simulink model "Einfache_Zustandsrueckfuehrung_nichtlinear"  (R2021b)
settings: Solver=VariableStepAuto  StartTime=0.0  StopTime=3  FixedStep=1/1e6  RelTol=1e-3
undefined symbols (not defined in the file): C_buck, k_LMI_1, L_buck, S, T_c, x_Ruhe
settings Model: Creator=basti  LastModifiedBy=basti

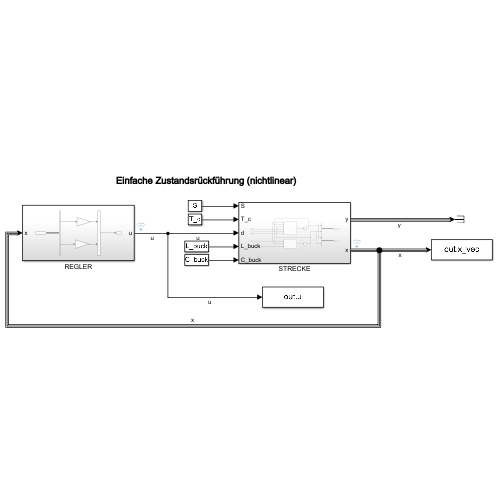
[thumbnail: Simulink's stored preview of the top-level diagram]
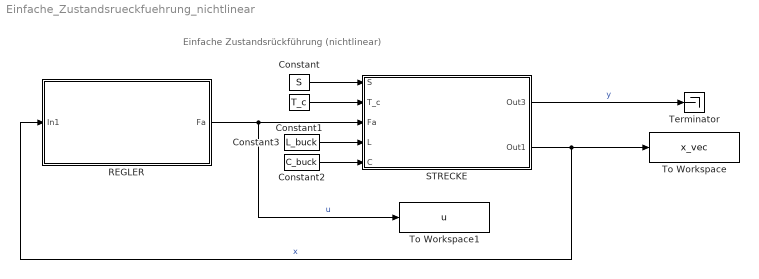
== system Einfache_Zustandsrueckfuehrung_nichtlinear ==
  note: Einfache Zustandsrückführung (nichtlinear)
  Constant : Constant  Value=S
  Constant1 : Constant  Value=T_c
  Constant2 : Constant  Value=C_buck
  Constant3 : Constant  Value=L_buck
  REGLER : Subsystem
  STRECKE : Subsystem
  Terminator : Terminator
  To Workspace : ToWorkspace  VariableName=x_vec  SaveFormat=Timeseries  SampleTime=-1
  To Workspace1 : ToWorkspace  VariableName=u  SaveFormat=Timeseries  SampleTime=-1
  wires:
  REGLER/1(Fa) -> STRECKE/3(Fa), To Workspace1/1  "u"
  STRECKE/1(Out3) -> Terminator/1  "y"
  STRECKE/2(Out1) -> REGLER/1(In1), To Workspace/1  "x"
  Constant3/1 -> STRECKE/4(L)
  Constant2/1 -> STRECKE/5(C)
  Constant/1 -> STRECKE/1(S)
  Constant1/1 -> STRECKE/2(T_c)

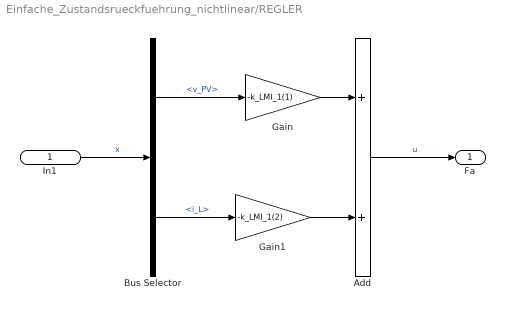
== system Einfache_Zustandsrueckfuehrung_nichtlinear/REGLER ==
  In1 : Inport
  Add : Sum
  Bus Selector : BusSelector  OutputSignals=v_PV,i_L
  Gain : Gain  Gain=-k_LMI_1(1)
  Gain1 : Gain  Gain=-k_LMI_1(2)
  Fa : Outport
  wires:
  Gain1/1 -> Add/2
  Gain/1 -> Add/1
  Add/1 -> Fa/1  "u"
  In1/1 -> Bus Selector/1  "x"
  Bus Selector/1 -> Gain/1  "<v_PV>"
  Bus Selector/2 -> Gain1/1  "<i_L>"

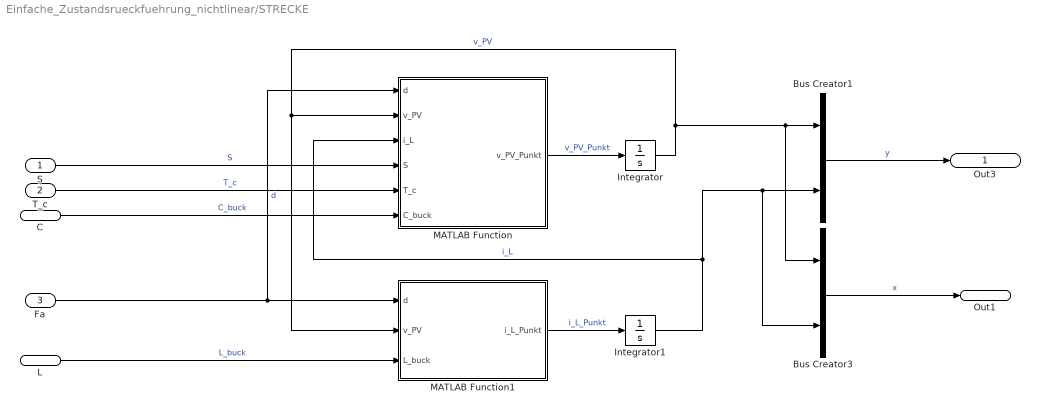
== system Einfache_Zustandsrueckfuehrung_nichtlinear/STRECKE ==
  S : Inport
  T_c : Inport  Port=2
  Fa : Inport  Port=3
  L : Inport  Port=4
  C : Inport  Port=5
  Bus Creator1 : BusCreator  Inputs=2
  Bus Creator3 : BusCreator  Inputs=2
  Integrator : Integrator  InitialCondition=x_Ruhe(1)*1.005
  Integrator1 : Integrator
  MATLAB Function : MATLAB Function  TreatAsAtomicUnit=on
  MATLAB Function1 : MATLAB Function  TreatAsAtomicUnit=on
  Out3 : Outport
  Out1 : Outport  Port=2
  wires:
  MATLAB Function1/1(i_L_Punkt) -> Integrator1/1  "i_L_Punkt"
  L/1 -> MATLAB Function1/3(L_buck)  "L_buck"
  T_c/1 -> MATLAB Function/5(T_c)  "T_c"
  C/1 -> MATLAB Function/6(C_buck)  "C_buck"
  Fa/1 -> MATLAB Function/1(d), MATLAB Function1/1(d)  "d"
  Integrator/1 -> Bus Creator1/1, Bus Creator3/1, MATLAB Function/2(v_PV), MATLAB Function1/2(v_PV)  "v_PV"
  S/1 -> MATLAB Function/4(S)  "S"
  Bus Creator1/1 -> Out3/1  "y"
  Integrator1/1 -> MATLAB Function/3(i_L), Bus Creator1/2, Bus Creator3/2  "i_L"
  MATLAB Function/1(v_PV_Punkt) -> Integrator/1  "v_PV_Punkt"
  Bus Creator3/1 -> Out1/1  "x"

== matlab function Einfache_Zustandsrueckfuehrung_nichtlinear/STRECKE/MATLAB Function1 ==
  data: d input; i_L_Punkt output; v_PV input; L_buck input
function i_L_Punkt = fcn(d, v_PV, L_buck)
    % Konstanten
    c = Konstanten();

    % Berechnung
    i_L_Punkt = 1/L_buck * v_PV * d - 1/L_buck * c.v_DC;

== matlab function Einfache_Zustandsrueckfuehrung_nichtlinear/STRECKE/MATLAB Function ==
  data: d input; v_PV_Punkt output; v_PV input; i_L input; S input; T_c input; C_buck input
% Eingänge

% Ausgänge

function v_PV_Punkt = fcn(d, v_PV, i_L, S, T_c, C_buck)
    % Konstanten
    c = Konstanten();

    % Berechnung
    v_oc = @(T_c) c.v_oc_STC * (1 + c.beta_T * (T_c - c.T_c_STC));                                      % für Modul
    i_ph = @(S, T_c) (S/c.S_STC) * c.i_ph_sc_STC * (1 + c.alpha_T * (T_c - c.T_c_STC));                 % für Modul
    i_s = @(S, T_c) (i_ph(S, T_c) - (v_oc(T_c)/c.R_h))/(exp(v_oc(T_c)/(c.A_n * c.v_T_STC)) - 1);        % für Modul
    i_d = @(x1, S, T_c) i_s(S, T_c) * (exp(x1/(c.N_s*c.v_T_STC * c.A_n)) - 1);                          % für Modul

    i_pv = @(x1, S, T_c) c.N_p * (i_ph(S, T_c) - i_d(x1, S, T_c) - x1/(c.N_s * c.R_h));

    % Ausgang
    v_PV_Punkt = 1/C_buck * i_pv(v_PV, S, T_c) - 1/C_buck * i_L * d;
